simulink model "pH_HyEq_model"  (R2017b)
settings: Solver=VariableStepAuto  StartTime=0.0  StopTime=60  MaxStep=0.01  RelTol=1e-3
values from neighbouring files (symbols this model uses):
  c_damping = 2    [pH_HyEq_init.m]
  J = 2000000    [pH_HyEq_init.m]
  K_d = 0*0.00002    (= 0)    [pH_HyEq_init.m]
  K_i = 0 * 0.00001    (= 0)    [pH_HyEq_init.m]
  K_i_sat = 1    [pH_HyEq_init.m]
  K_p = 0.3    [pH_HyEq_init.m]
  pH_inputs = [ ... (first row only)    [pH_HyEq_init.m]
  pump_limiter = 1    [pH_HyEq_init.m]
  rule = 1    [pH_HyEq_init.m]
  T = 2000000    [pH_HyEq_init.m]
  T_pH_star = 2    [pH_HyEq_init.m]
  x0 = [ ... (first row only)    [pH_HyEq_init.m]    (also in pH_HyEq_plot.m)
libraries: simulink x3
settings Model: Creator=jaidenking  LastModifiedBy=jaidenking

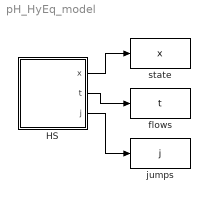
== system pH_HyEq_model ==
  HS : Subsystem  LoadFcn=set_param(gcb,'LinkStatus','none')  InitFcn=pH_HyEq_init  StopFcn=pH_HyEq_plot
      settings: CopyFcn=|
      | set_param(gcb,'LinkStatus','none'),
      | set_param(gcs, 'MaxStep', 'MaxStep', 'RelTol', 'RelTol','Stop time', 'T')
      mask Display:
      | image(imread('Hcal.jpg'))
      | %plot([5 20 20 5 5],[5 5 20 20 5])
      | %text(8,13,'HyEq_mdl')
      | port_label('output', 1, 'x')
      | port_label('output', 2, 't')
      | port_label('output', 3, 'j')
  flows : ToWorkspace  VariableName=t  SampleTime=-1
  jumps : ToWorkspace  VariableName=j  SampleTime=-1
  state : ToWorkspace  VariableName=x  SampleTime=-1
  wires:
  HS/3(j) -> jumps/1
  HS/2(t) -> flows/1
  HS/1(x) -> state/1

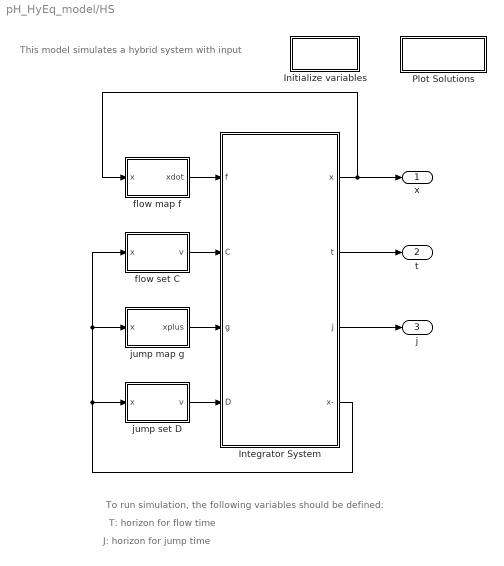
== system pH_HyEq_model/HS ==
  note: J: horizon for jump time
  note: T: horizon for flow time
  note: To run simulation, the following variables should be defined:
  note: This model simulates a hybrid system with input
  Initialize variables : Subsystem  Priority=-10
      settings: OpenFcn=pH_HyEq_init
      mask Display: disp('Double Click\n to Initialize')
  Integrator System : Subsystem  Priority=2  mask(Hybrid Integrator){T=T, J=J, x0=x0}
      mask prompts: T "Flow Horizon"; J "Jump Horizon"; x0 "Initial Condition"
      mask help:
      | This block integrates the state of the hybrid system defined by the flow map f (first input), the flow set C (second input), the jump map g (third input) and the jump set D (fourth input).
      | Starting from the initial condition x0 (last mask parameter), the system's state x evolves continuously within the set C, according to f(x,u), but is also subject to jumps within D, according to g(x,u).
      | The block also stops the simulation when the time t is greater than the flow horizon T (first mask parameter), or when the number of jumps j is greater than the jump horizon J (second mask parameter).
      | The outputs of the blocks are respectively x(t), t, j, x(t-).
      mask Help:
      | This block integrates the state of the hybrid system defined by the flow map f (first input), the flow set C (second input), the jump map g (third input) and the jump set D (fourth input).
      | <br>
      | Starting from the initial condition x0 (last mask parameter), the system's state x evolves continuously within the set C, according to f(x,u), but is also subject to jumps within D, according to g(x,u).
      | <br>
      | The block also stops the simulation when the time t is greater than the flow horizon T (first mask parameter), or when the number of jumps j is greater than the jump horizon J (second mask parameter).
      | <br>
      | The outputs of the blocks are respectively x(t), t, j, x(t-).
      | <br>
      | You can right click on the block and "Look under mask" to see what's inside the block.
      | Finally, refer to the manual (HybridSimulator_vXX.pdf) for more detailed information on how this hybrid simulator works.
  Plot Solutions : Subsystem
      settings: OpenFcn=pH_HyEq_plot
      mask Display: disp('Double Click to\n Plot Solutions')
  flow map f : MATLAB Function  TreatAsAtomicUnit=on
  flow set C : MATLAB Function  TreatAsAtomicUnit=on
  jump map g : MATLAB Function  Priority=2  TreatAsAtomicUnit=on
  jump set D : MATLAB Function  TreatAsAtomicUnit=on
  x : Outport
  t : Outport  Port=2
  j : Outport  Port=3
  wires:
  jump map g/1(xplus) -> Integrator System/3(g)
  jump set D/1(v) -> Integrator System/4(D)
  Integrator System/3(j) -> j/1
  Integrator System/2(t) -> t/1
  flow set C/1(v) -> Integrator System/2(C)
  Integrator System/1(x) -> x/1, flow map f/1(x)
  Integrator System/4(x-) -> jump set D/1(x), flow set C/1(x), jump map g/1(x)
  flow map f/1(xdot) -> Integrator System/1(f)

== system pH_HyEq_model/HS/Initialize variables ==

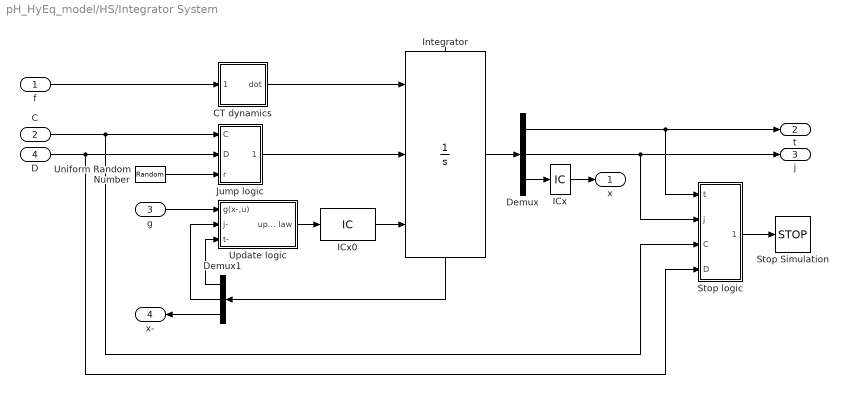
== system pH_HyEq_model/HS/Integrator System ==
  f : Inport
  C : Inport  Port=2
  g : Inport  Port=3
  D : Inport  Port=4
  CT dynamics : Subsystem
  Demux : Demux  Outputs=[1 1 -1]
  Demux1 : Demux  Outputs=[1 1 -1]
  ICx : InitialCondition  Value=x0
  ICx0 : InitialCondition  Value=[0; 0; x0(:)]
  Integrator : Integrator  ExternalReset=level hold  InitialConditionSource=external  ShowStatePort=on  ZeroCross=off
  Jump logic : Subsystem
  Stop Simulation : Stop
  Stop logic : Subsystem
  Uniform Random Number : UniformRandomNumber  Minimum=0  Seed=abs(floor(100*rand))  SampleTime=0
  Update logic : Subsystem
  x : Outport
  t : Outport  Port=2
  j : Outport  Port=3
  x- : Outport  Port=4
  wires:
  ICx0/1 -> Integrator/3
  ICx/1 -> x/1
  Demux/3 -> ICx/1
  Integrator/State -> Demux1/1
  Demux/2 -> j/1, Stop logic/2(j)
  Demux/1 -> t/1, Stop logic/1(t)
  Update logic/1(update law) -> ICx0/1
  CT dynamics/1(dot) -> Integrator/1
  Stop logic/1(stop) -> Stop Simulation/1
  Integrator/1 -> Demux/1
  C/1 -> Stop logic/3(C), Jump logic/1(C)
  D/1 -> Stop logic/4(D), Jump logic/2(D)
  f/1 -> CT dynamics/1(f(x,u))
  Demux1/3 -> x-/1
  Jump logic/1(jump) -> Integrator/2
  Uniform Random Number/1 -> Jump logic/3(r)
  g/1 -> Update logic/1(g(x-,u))
  Demux1/1 -> Update logic/3(t-)
  Demux1/2 -> Update logic/2(j-)

== system pH_HyEq_model/HS/Plot Solutions ==

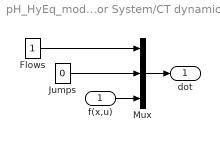
== system pH_HyEq_model/HS/Integrator System/CT dynamics ==
  f(x,u) : Inport
  Flows : Constant
  Jumps : Constant  Value=0
  Mux : Mux  Inputs=[1 1 -1]
  dot : Outport
  wires:
  Jumps/1 -> Mux/2
  Flows/1 -> Mux/1
  Mux/1 -> dot/1
  f(x,u)/1 -> Mux/3

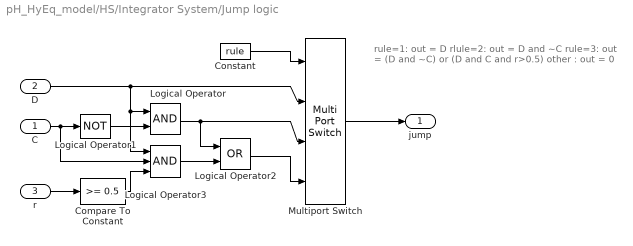
== system pH_HyEq_model/HS/Integrator System/Jump logic ==
  note: rule=1:  out = D
      | rlule=2: out = D and ~C
      | rule=3:  out = (D and ~C)  or (D and C and r>0.5)
      | other :  out = 0
  C : Inport
  D : Inport  Port=2
  r : Inport  Port=3
  Compare To Constant : simulink/Logic and Bit Operations/Compare To Constant  relop=>=  const=0.5  OutDataTypeStr=uint8
  Constant : Constant  Value=rule
  Logical Operator : Logic  AllPortsSameDT=off  OutDataTypeStr=boolean
  Logical Operator1 : Logic  Operator=NOT  Inputs=1  AllPortsSameDT=off  OutDataTypeStr=boolean
  Logical Operator2 : Logic  Operator=OR  AllPortsSameDT=off  OutDataTypeStr=boolean
  Logical Operator3 : Logic  Inputs=3  AllPortsSameDT=off  OutDataTypeStr=boolean
  Multiport Switch : MultiPortSwitch
  jump : Outport
  wires:
  Constant/1 -> Multiport Switch/1
  D/1 -> Logical Operator3/1, Logical Operator/1, Multiport Switch/2
  r/1 -> Compare To Constant/1
  C/1 -> Logical Operator3/2, Logical Operator1/1
  Logical Operator1/1 -> Logical Operator/2
  Logical Operator/1 -> Multiport Switch/3, Logical Operator2/1
  Logical Operator2/1 -> Multiport Switch/4
  Multiport Switch/1 -> jump/1
  Compare To Constant/1 -> Logical Operator3/3
  Logical Operator3/1 -> Logical Operator2/2

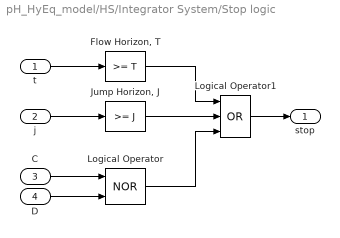
== system pH_HyEq_model/HS/Integrator System/Stop logic ==
  t : Inport
  j : Inport  Port=2
  C : Inport  Port=3
  D : Inport  Port=4
  "Flow Horizon, T" : simulink/Logic and Bit Operations/Compare To Constant  relop=>=  const=T  OutDataTypeStr=uint8  ZeroCross=off
  "Jump Horizon, J" : simulink/Logic and Bit Operations/Compare To Constant  relop=>=  const=J  OutDataTypeStr=uint8  ZeroCross=off
  Logical Operator : Logic  Operator=NOR  AllPortsSameDT=off  OutDataTypeStr=boolean
  Logical Operator1 : Logic  Operator=OR  Inputs=3  AllPortsSameDT=off  OutDataTypeStr=boolean
  stop : Outport
  wires:
  "Flow Horizon, T"/1 -> Logical Operator1/1
  "Jump Horizon, J"/1 -> Logical Operator1/2
  Logical Operator/1 -> Logical Operator1/3
  D/1 -> Logical Operator/2
  t/1 -> "Flow Horizon, T"/1
  j/1 -> "Jump Horizon, J"/1
  C/1 -> Logical Operator/1
  Logical Operator1/1 -> stop/1

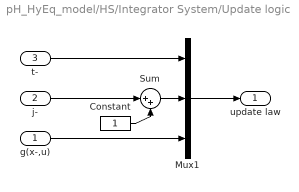
== system pH_HyEq_model/HS/Integrator System/Update logic ==
  g(x-,u) : Inport
  j- : Inport  Port=2
  t- : Inport  Port=3
  Constant : Constant
  Mux1 : Mux  Inputs=[1 1 -1]
  Sum : Sum  Inputs=|++
  update law : Outport
  wires:
  Sum/1 -> Mux1/2
  Mux1/1 -> update law/1
  j-/1 -> Sum/1
  g(x-,u)/1 -> Mux1/3
  t-/1 -> Mux1/1
  Constant/1 -> Sum/2

== matlab function pH_HyEq_model/HS/flow map f ==
  data: x input; xdot output; K_p parameter; K_d parameter; c_damping parameter
function xdot = f(x, K_p, K_d, c_damping)
%--------------------------------------------------------------------------
% Matlab M-file Project: HyEQ Toolbox @  Hybrid Systems Laboratory (HSL), 
% https://hybrid.soe.ucsc.edu/software
% http://hybridsimulator.wordpress.com/
%--------------------------------------------------------------------------
% Project: Simulation of a hybrid system
% Description: Flow map
%--------------------------------------------------------------------------
%--------------------------------------------------------------------------
%   See also HYEQSOLVER, PLOTARC, PLOTARC3, PLOTFLOWS, PLOTHARC,
%   PLOTHARCCOLOR, PLOTHARCCOLOR3D, PLOTHYBRIDARC, PLOTJUMPS.
%   Copyright @ Hybrid Systems Laboratory (HSL),
%   Revision: 0.0.0.3 Date: 05/20/2015 3:42:00

%{
x0 = [
   0;              % 1 continuous time 
   0;              % 2 discrete time
   pH_inputs(1,3); % 3 time when the previous drop of pH up/down was added
   pH_inputs(1,3); % 4 Steady-state pH
   pH_inputs(1,3); % 5 Previous steady-state pH
   pH_inputs(1,3); % 6 Current pH
   2;              % 7 Next pH input 
   1;              % 8 Mixing coefficient
   pH_inputs(1,1); % 9 Solution volume
   pH_inputs(1,2); % 10 Solution density
   0;              % 11 pH velocity
   0;              % 12 Steady-state velocity
   4;              % 13 pump timer
   1;              % 14 pump state
   0;              % 15 measured pH
   T_pH_star       % 16 pH Sensor Timer
   0;              % 17 Integrated error
];
%}

%{
pumpActuation =  K_p*(8-x(15)) - K_d*x(12);
if(pumpActuation > 0 && x(12) >= 1) 
    pumpActuation = 0;
elseif(pumpActuation < 0 && x(12) <= -1)
    pumpActuation = 0;
end
%}

xdot = [
   1; % Continuous time
   0;
   0;
   x(12); % Stead-state pH. "Force" of the mass-spring-damper system. Changes based on pump speed
   0;
   x(11); % Current pH
   0;
   0;
   0;
   0;
   x(4) - c_damping*x(11) - 1*x(6); % pH speed. "Velocity" of the mass-spring-damper system.
   0; %pumpActuation;
   x(14);
   0;
   0;
   x(18);
   0;
   0;
];

== matlab function pH_HyEq_model/HS/flow set C ==
  data: x input; v output
function v  = C(x) 
%--------------------------------------------------------------------------
% Matlab M-file Project: HyEQ Toolbox @  Hybrid Systems Laboratory (HSL), 
% https://hybrid.soe.ucsc.edu/software
% http://hybridsimulator.wordpress.com/
%--------------------------------------------------------------------------
% Project: Simulation of a hybrid system
% Description: Flow set
%--------------------------------------------------------------------------
%--------------------------------------------------------------------------
%   See also HYEQSOLVER, PLOTARC, PLOTARC3, PLOTFLOWS, PLOTHARC,
%   PLOTHARCCOLOR, PLOTHARCCOLOR3D, PLOTHYBRIDARC, PLOTJUMPS.
%   Copyright @ Hybrid Systems Laboratory (HSL),
%   Revision: 0.0.0.3 Date: 05/20/2015 3:42:00
%
% Check on flow conditions
% E.g.,
% if (x(1) >= u(1))  % flow condition
%     v = 1;  % report flow
% else
%     v = 0;   % do not report flow
% end

v = 1;

== matlab function pH_HyEq_model/HS/jump map g ==
  settings: updateMethod=DISCRETE
  data: x input; xplus output size=18; pH_inputs parameter; T_pH_star parameter; K_p parameter; K_d parameter; K_i parameter; K_i_sat parameter; pump_limiter parameter
function xplus = g(x,pH_inputs,T_pH_star,K_p, K_d, K_i, K_i_sat, pump_limiter)
%--------------------------------------------------------------------------
% Matlab M-file Project: HyEQ Toolbox @  Hybrid Systems Laboratory (HSL), 
% https://hybrid.soe.ucsc.edu/software
% http://hybridsimulator.wordpress.com/
%--------------------------------------------------------------------------
% Project: Simulation of a hybrid system
% Description: Jump map
%--------------------------------------------------------------------------
%--------------------------------------------------------------------------
%   See also HYEQSOLVER, PLOTARC, PLOTARC3, PLOTFLOWS, PLOTHARC,
%   PLOTHARCCOLOR, PLOTHARCCOLOR3D, PLOTHYBRIDARC, PLOTJUMPS.
%   Copyright @ Hybrid Systems Laboratory (HSL),
%   Revision: 0.0.0.3 Date: 05/20/2015 3:42:00

%{
pH_inputs = [
   % volume, density, pH, time
];
x0 = [
   0;              % 1 continuous time 
   0;              % 2 discrete time
   pH_inputs(1,3); % 3 time when the previous drop of pH up/down was added
   8; %pH_inputs(1,3); % 4 Steady-state pH
   pH_inputs(1,3); % 5 Previous steady-state pH
   pH_inputs(1,3); % 6 Current pH
   2;              % 7 Next pH input 
   1;              % 8 Mixing coefficient
   pH_inputs(1,1); % 9 Solution volume
   pH_inputs(1,2); % 10 Solution density
   0;              % 11 pH velocity
   0;              % 12 Steady-state velocity
   4;              % 13 pump timer
   1;              % 14 pump state
   pH_inputs(1,3); % 15 measured pH
   T_pH_star       % 16 pH Sensor Timer
   0;              % 17 Integrated error
];
%}
xplus = x(:);

if(x(13)<=0)
   % pump timer expired
   xplus(12) = 0; % Shut off pump
   xplus(14) = 0; % Stop pump timer
   xplus(13) = 1; % Reset pump timer
   xplus(18) = -1; % Start sensor timer
end
if(x(16)<=0)
   % sensor timer expired
   xplus(18) = 0; % Stop sensor timer
   xplus(16) = T_pH_star; % Reset sensor timer
   xplus(14) = -1; % Start pump timer
   xplus(12) = pump_limiter; % Start pump
   xplus(15) = x(6);
   err = 8-x(6);
   if(err<0)
       xplus(12) = xplus(12) * -1;
   end
   xplus(13) = abs(err) * K_p; % Set pump timer
end

%{
if(x(16)<=0)
    % Discrete time control algorithm
    err = 8-x(6);
    vel = (x(6)-x(15))/T_pH_star;
    xplus(17) = x(17) + K_i * err;
    xplus(17) = max([min([xplus(17) K_i_sat]) -K_i_sat]);
    
    pumpActuation =  K_p*(err) + K_d*(-vel) + xplus(17);
    if(pumpActuation > 0 && x(12) >= pump_limiter) 
        pumpActuation = 0;
    elseif(pumpActuation < 0 && x(12) <= -pump_limiter)
        pumpActuation = 0;
    end
 
   xplus(12) = x(12) + pumpActuation;
   xplus(12) = min([max([xplus(12) -pump_limiter]) pump_limiter]);
   xplus(15) = x(6);
   xplus(16) = T_pH_star;
   
   
end
%}

== matlab function pH_HyEq_model/HS/jump set D ==
  data: x input; v output; pH_inputs parameter
function v  = D(x,pH_inputs) 
%--------------------------------------------------------------------------
% Matlab M-file Project: HyEQ Toolbox @  Hybrid Systems Laboratory (HSL), 
% https://hybrid.soe.ucsc.edu/software
% http://hybridsimulator.wordpress.com/
%--------------------------------------------------------------------------
% Project: Simulation of a hybrid system
% Description: Jump set
%--------------------------------------------------------------------------
%--------------------------------------------------------------------------
%   See also HYEQSOLVER, PLOTARC, PLOTARC3, PLOTFLOWS, PLOTHARC,
%   PLOTHARCCOLOR, PLOTHARCCOLOR3D, PLOTHYBRIDARC, PLOTJUMPS.
%   Copyright @ Hybrid Systems Laboratory (HSL),
%   Revision: 0.0.0.3 Date: 05/20/2015 3:42:00
%
% Check on jump conditions
% % E.g.,
% if (x(1) <= u(1)) && (x(2) <= 0)  % jump condition
%     v = 1;  % report jump
% else
%     v = 0;   % do not report jump
% end

%{
x0 = [
   0;              % 1 continuous time 
   0;              % 2 discrete time
   pH_inputs(1,3); % 3 time when the previous drop of pH up/down was added
   pH_inputs(1,3); % 4 Steady-state pH
   pH_inputs(1,3); % 5 Previous steady-state pH
   pH_inputs(1,3); % 6 Current pH
   2;              % 7 Next pH input 
   1;              % 8 Mixing coefficient
   pH_inputs(1,1); % 9 Solution volume
   pH_inputs(1,2); % 10 Solution density
   0;              % 11 pH velocity
   0;              % 12 Steady-state velocity
   4;              % 13 pump timer
   1;              % 14 pump state
   0;              % 15 measured pH
   T_pH_star       % 16 pH Sensor Timer
];
%}
v = 0;

if(x(13)<=0)
    % pump timer expired
    v = 1; 
end
if(x(16)<=0)
    % pH sensor timer expired
    v = 1;
end
